simulink model "ref_model"  (R2022b)
settings: Solver=ode5  StartTime=0.0  StopTime=10.0  FixedStep=.02  RelTol=1e-3
settings Model: Creator=hp_desktop  LastModifiedBy=hp_desktop
settings ModelReferenceCC: UseModelRefSolver=on

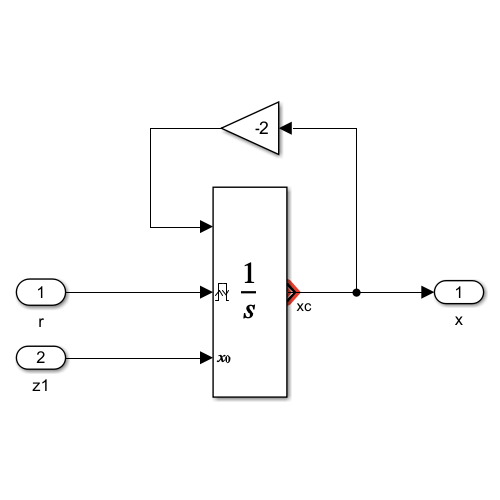
[thumbnail: Simulink's stored preview of the top-level diagram]
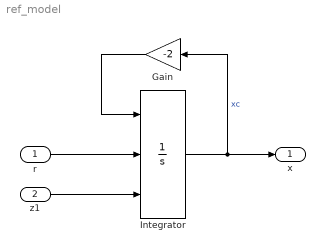
== system ref_model ==
  r : Inport
  z1 : Inport  Port=2
  Gain : Gain  Gain=-2
  Integrator : Integrator  ExternalReset=either  InitialConditionSource=external
  x : Outport
  wires:
  z1/1 -> Integrator/3
  r/1 -> Integrator/2
  Integrator/1 -> x/1, Gain/1  "xc"
  Gain/1 -> Integrator/1
